simulink model "Muscle-Stretch-Reflex-Analysis_simulation"  (R2024b)
settings: Solver=VariableStepAuto  StartTime=0.0  StopTime=10.0  RelTol=1e-3
settings Model: Creator=nafis  LastModifiedBy=nafis
settings SolverCC: DateTimeAtSimulationTimeZero=[]

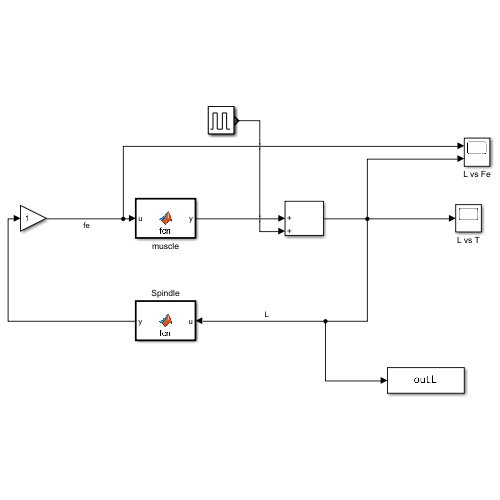
[thumbnail: Simulink's stored preview of the top-level diagram]
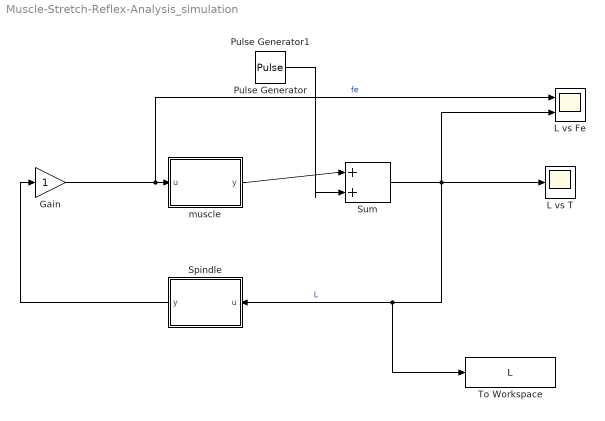
== system Muscle-Stretch-Reflex-Analysis_simulation ==
  Gain : Gain
  L vs Fe : Scope  NumInputPorts=2
  L vs T : Scope
  Pulse Generator : DiscretePulseGenerator  PulseType=Time based  Period=15  PulseWidth=0.75
  Pulse Generator1 : DiscretePulseGenerator  PulseType=Time based  Period=10  PulseWidth=5
  Spindle : MATLAB Function  TreatAsAtomicUnit=on
  Sum : Sum  Inputs=|++
  To Workspace : ToWorkspace  VariableName=L  SaveFormat=Timeseries  SampleTime=-1
  muscle : MATLAB Function  TreatAsAtomicUnit=on
  wires:
  Gain/1 -> L vs Fe/1, muscle/1(u)  "fe"
  muscle/1(y) -> Sum/1
  Pulse Generator1/1 -> Sum/2
  Sum/1 -> L vs Fe/2, To Workspace/1, Spindle/1(u), L vs T/1  "L"
  Spindle/1(y) -> Gain/1

== matlab function Muscle-Stretch-Reflex-Analysis_simulation/muscle ==
  data: u input; y output
function y = fcn(u)

y = 1-u^5/(0.5^5+u^5);

== matlab function Muscle-Stretch-Reflex-Analysis_simulation/Spindle ==
  data: u input; y output
function y = fcn(u)

y = (6/10)*u*exp(5*u/10);
